simulink model "bilibiliExample"  (R2019a)
settings: Solver=FixedStepAuto  StartTime=0.0  StopTime=15  FixedStep=0.001  RelTol=1e-3
PreLoadFcn:
  | % 创建变量
  | degConv = 180/pi;
settings Model: PauseTimes=0  OrderedModelArguments=off  Creator=FJJ  LastModifiedBy=FJJ
settings DataIOCC: ExternalInput=bilibiliExData1.getElement(1)  LoadExternalInput=on

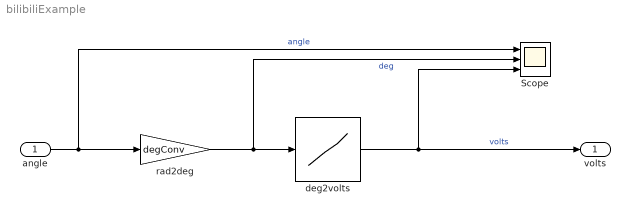
== system bilibiliExample ==
  angle : Inport  Unit=rad
  Scope : Scope  NumInputPorts=3
  deg2volts : Lookup_n-D  NumberOfTableDimensions=1  BreakpointsForDimension1=[0, 90]  Table=[0.5 4.5]  ExtrapMethod=Clip  InternalRulePriority=Speed  RndMeth=Simplest  InputSameDT=on
  rad2deg : Gain  Gain=degConv
  volts : Outport
  wires:
  angle/1 -> Scope/1, rad2deg/1  "angle"
  rad2deg/1 -> Scope/2, deg2volts/1  "deg"
  deg2volts/1 -> Scope/3, volts/1  "volts"
